simulink model "Simu_FIR"  (R2022b)
settings: Solver=ode4  StartTime=0.0  StopTime=simu.hor  FixedStep=simu.dt  RelTol=1e-3  EnableMultiTasking=on
values from neighbouring files (symbols this model uses):
  filtre = rmfield(filtre,'NomAlgo')    [choix_simu.m]
  simu = simulation    [choix_simu.m]
undefined symbols (not defined in the file or in its folder): source
libraries: simulink x4
settings Model: Creator=mouyon  LastModifiedBy=mathe
settings SolverCC: AlgebraicLoopSolver=TrustRegion
settings DataIOCC: LimitDataPoints=on  ReturnWorkspaceOutputs=off
settings OptimizationCC: LifeSpan=inf
settings DebuggingCC: ArtificialAlgebraicLoopMsg=none  UnconnectedInputMsg=warning  UnconnectedOutputMsg=warning  UnconnectedLineMsg=warning  AllowSymbolicDim=off  SFUnexpectedBacktrackingDiag=warning  SFNoUnconditionalDefaultTransitionDiag=warning  SFExecutionAtInitializationDiag=none  SFMachineParentedDataDiag=warning  ArithmeticOperatorsInVariantConditions=warning
settings ModelReferenceCC: EnableRefExpFcnMdlSchedulingChecks=on  PropagateSignalLabelsOutOfModel=off
settings SFSimCC: SimUseLocalCustomCode=off  CustomCodeUndefinedFunction=UseInterfaceOnly
settings RTWCC: RTWUseLocalCustomCode=off
settings CodeAppCC: StateflowObjectComments=on
settings GRTTargetCC: TargetLangStandard=C89/C90 (ANSI)
settings ConfigComp: CovMetricSettings=dw  CovSaveCumulativeToWorkspaceVar=on  CovSaveSingleToWorkspaceVar=on  CovExternalEMLEnable=off

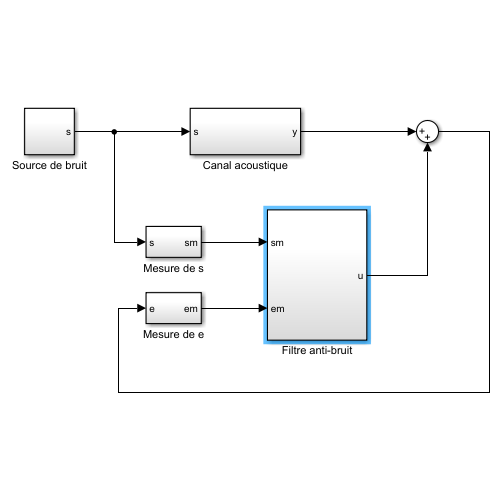
[thumbnail: Simulink's stored preview of the top-level diagram]
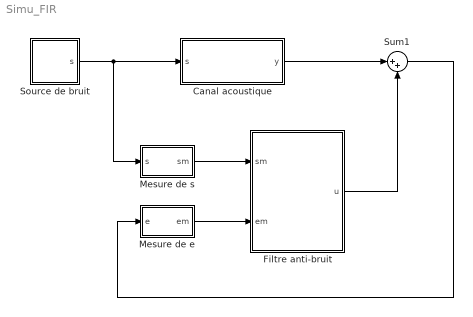
== system Simu_FIR ==
  Canal acoustique : Subsystem
  Filtre anti-bruit : Subsystem
  Mesure de e : Subsystem
  Mesure de s : Subsystem
  Source de bruit : Subsystem
  Sum1 : Sum  Inputs=|++
  wires:
  Source de bruit/1(s) -> Canal acoustique/1(s), Mesure de s/1(s)
  Mesure de s/1(sm) -> Filtre anti-bruit/1(sm)
  Mesure de e/1(em) -> Filtre anti-bruit/2(em)
  Sum1/1 -> Mesure de e/1(e)
  Filtre anti-bruit/1(u) -> Sum1/2
  Canal acoustique/1(y) -> Sum1/1

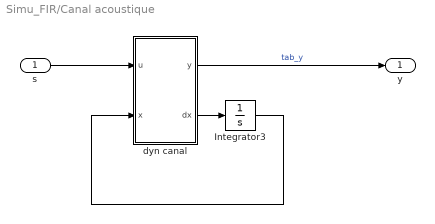
== system Simu_FIR/Canal acoustique ==
  s : Inport
  Integrator3 : Integrator  InitialCondition=[0;0]
  dyn canal : MATLAB Function  TreatAsAtomicUnit=on
  y : Outport
  wires:
  s/1 -> dyn canal/1(u)
  dyn canal/1(y) -> y/1  "tab_y"
  dyn canal/2(dx) -> Integrator3/1
  Integrator3/1 -> dyn canal/2(x)

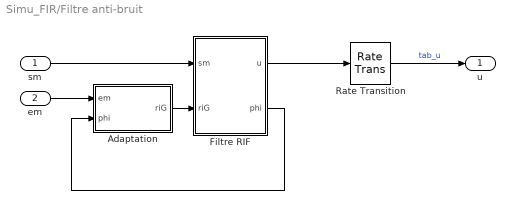
== system Simu_FIR/Filtre anti-bruit ==
  sm : Inport
  em : Inport  Port=2
  Adaptation : Subsystem
  Filtre RIF : Subsystem
  Rate Transition : RateTransition  OutPortSampleTime=simu.dt
  u : Outport
  wires:
  Rate Transition/1 -> u/1  "tab_u"
  em/1 -> Adaptation/1(em)
  Filtre RIF/1(u) -> Rate Transition/1
  sm/1 -> Filtre RIF/1(sm)
  Adaptation/1(riG) -> Filtre RIF/2(riG)
  Filtre RIF/2(phi) -> Adaptation/2(phi)

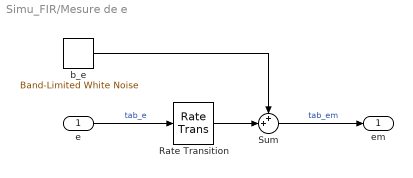
== system Simu_FIR/Mesure de e ==
  e : Inport
  Rate Transition : RateTransition  OutPortSampleTime=filtre.dt
  Sum : Sum  Inputs=++|
  b_e : simulink/Sources/Band-Limited White Noise  Cov=(simu.sigbe)^2  Ts=filtre.dt  seed=[23341]
  em : Outport
  wires:
  e/1 -> Rate Transition/1  "tab_e"
  b_e/1 -> Sum/1
  Sum/1 -> em/1  "tab_em"
  Rate Transition/1 -> Sum/2

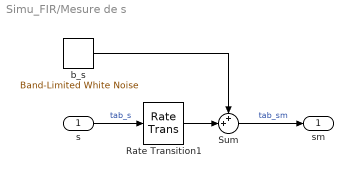
== system Simu_FIR/Mesure de s ==
  s : Inport
  Rate Transition1 : RateTransition  OutPortSampleTime=filtre.dt
  Sum : Sum  Inputs=++|
  b_s : simulink/Sources/Band-Limited White Noise  Cov=(simu.sigbs)^2  Ts=filtre.dt  seed=[23341]
  sm : Outport
  wires:
  b_s/1 -> Sum/1
  Sum/1 -> sm/1  "tab_sm"
  Rate Transition1/1 -> Sum/2
  s/1 -> Rate Transition1/1  "tab_s"

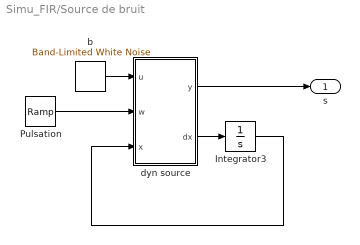
== system Simu_FIR/Source de bruit ==
  Integrator3 : Integrator  InitialCondition=[0;0]
  Pulsation : simulink/Sources/Ramp  slope=(source.wf-source.wi)/simu.hor  start=0  InitialOutput=source.wi
  b : simulink/Sources/Band-Limited White Noise  Cov=1  Ts=simu.dt  seed=[23341]
  dyn source : MATLAB Function  TreatAsAtomicUnit=on
  s : Outport
  wires:
  dyn source/2(dx) -> Integrator3/1
  Integrator3/1 -> dyn source/3(x)
  Pulsation/1 -> dyn source/2(w)
  dyn source/1(y) -> s/1
  b/1 -> dyn source/1(u)

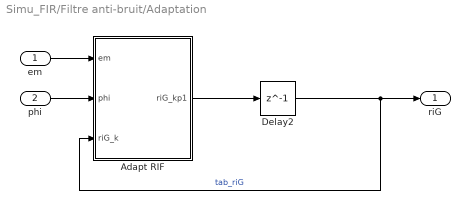
== system Simu_FIR/Filtre anti-bruit/Adaptation ==
  em : Inport
  phi : Inport  Port=2
  Adapt RIF : MATLAB Function  TreatAsAtomicUnit=on
  Delay2 : Delay  DelayLength=1  InitialCondition=filtre.riG_ini  SampleTime=filtre.dt
  riG : Outport
  wires:
  em/1 -> Adapt RIF/1(em)
  phi/1 -> Adapt RIF/2(phi)
  Adapt RIF/1(riG_kp1) -> Delay2/1
  Delay2/1 -> Adapt RIF/3(riG_k), riG/1  "tab_riG"

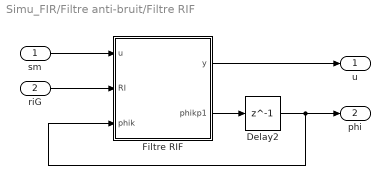
== system Simu_FIR/Filtre anti-bruit/Filtre RIF ==
  sm : Inport
  riG : Inport  Port=2
  Delay2 : Delay  DelayLength=1  InitialCondition=zeros(filtre.Nx,1)  SampleTime=filtre.dt
  Filtre RIF : MATLAB Function  TreatAsAtomicUnit=on
  u : Outport
  phi : Outport  Port=2
  wires:
  sm/1 -> Filtre RIF/1(u)
  riG/1 -> Filtre RIF/2(RI)
  Filtre RIF/1(y) -> u/1
  Filtre RIF/2(phikp1) -> Delay2/1
  Delay2/1 -> Filtre RIF/3(phik), phi/1

== matlab function Simu_FIR/Source de bruit/dyn source ==
  data: u input size=1; y output size=1; w input size=1; x input size=[2,1]; dx output size=[2,1]; source parameter
function [y,dx] = dyn_source(u,w,x,source)

%-----------------------------------------------------------
% bruit acoustique
%-----------------------------------------------------------
% u :	bruit blanc normalisé
% w :	pulsation instantannée
% x :	vecteur d'état
% source.xi :  amortissement
% 
% y :	bruit acoustique
% dx :	dérivée du vecteur  d'état
%-----------------------------------------------------------

xi = source.xi;

dx = zeros(2,1);
dx(1,1) = x(2,1);
dx(2,1) = -w*w*x(1,1) - 2*xi*w*x(2,1) + w*w*u;

y = x(1,1);

== matlab function Simu_FIR/Filtre anti-bruit/Adaptation/Adapt RIF ==
  settings: updateMethod=DISCRETE  sampleTime=filtre.dt
  data: riG_kp1 output size=[filtre.Nx,1]; em input size=1; phi input size=[filtre.Nx,1]; riG_k input size=[filtre.Nx,1]; filtre parameter
function riG_kp1  = Adapt_rif(em,phi,riG_k,filtre)

% [riG_kp1] = Adapt_rif(em,phi,riG_k,filtre);
%-----------------------------------------------------------------------
% Adapatation d'un filtre RIF
%-----------------------------------------------------------------------
% em :      signal à minimise
% phi :     régresseur (vecteur d'état du filtre)
% riG_k :	réponse impulsionnelle du filtre (paramètres du filtre)
% filtre.NumAlgo :	numéro de l'algorithme d'adaptation
% filtre.mu :       pas de l'algorithme d'adaptation
% 
% riG_kp1 :	réponse impulsionnelle du filtre mise à jour
%-----------------------------------------------------------------------
% NumAlgo : 
% 0 = sans d'adaptation
% 1 = algorithme du NLMS
% 2 = algorithme du LMS
% 3 = algorithme du RLS
%-----------------------------------------------------------------------

% Initialisations
NumAlgo = filtre.NumAlgo;
mu      = filtre.mu;
riG_kp1 = riG_k;

eps = 1e-8;

switch NumAlgo
    case 0
        % Pas d'adaptation
        riG_kp1 = riG_k;
        
    case 1
        % Adaptation par gradient stochastique normalisé
        % fprintf('NLMS - Algorithme non codé!!!\n');
        riG_kp1 = riG_k - (mu/2) * phi * em / (phi'*phi+eps);
        
    case 2
        % Adaptation par gradient stochastique
%         fprintf('LMS - Algorithme non codé!!!\n');
        riG_kp1 = riG_k - 2 * mu * phi * em;
        
    case 3
        % Adaptation par moindres carrés récursifs
%         fprintf('RLS - Algorithme non codé!!!\n');
        Hk = 2 * phi' * phi + eps;
        gk = - 2 * phi * em;
        riG_kp1 = riG_k + mu * inv(Hk) * gk;

    otherwise
        fprintf('Algorithme non codé!!!\n');
        riG_kp1 = riG_k;
end;

== matlab function Simu_FIR/Canal acoustique/dyn canal ==
  data: u input size=1; x input size=[2,1]; y output size=1; canal parameter; dx output size=[2,1]
function [y,dx] = dyn_canal(u,x,canal)

%-----------------------------------------------------------
% canal acoustique
%-----------------------------------------------------------
% u :   bruit émis par la source
% canal.w  :	pulsation
% canal.xi :	amortissement
% canal.g  :    gain 
%
% y :   bruit transmis par le canal
% dx :	dérivée du vecteur  d'état
%-----------------------------------------------------------

w  = canal.w;
xi = canal.xi;
g  = canal.g;

dx = zeros(2,1);
dx(1,1) = x(2,1);
dx(2,1) = -w*w*x(1,1) - 2*xi*w*x(2,1) + w*w*u;

y = g * x(1,1);

== matlab function Simu_FIR/Filtre anti-bruit/Filtre RIF/Filtre RIF ==
  settings: updateMethod=DISCRETE  sampleTime=filtre.dt
  data: y output size=1; u input size=1; RI input size=[filtre.Nx,1]; phikp1 output size=[filtre.Nx,1]; phik input size=[filtre.Nx,1]
function [y,phikp1] = filtre_rif(u,RI,phik)

% [y,phikp1] = filtre_rif(u,RI,phik);
%-----------------------------------------------------------------------
% Filtre RIF
%-----------------------------------------------------------------------
% u :       signal à filtrer
% RI :      réponse impulsionnelle du filtre 
% phik :	régresseur (vecteur d'état)
% 
% y :       signal filtré
% phikp1 :	régresseur mis à jour
%-----------------------------------------------------------------------

% Sortie
y = phik'*RI;

% Integration des etats
phikp1 = [u ; phik(1:end-1,1)];
